simulink model "figure11_62"  (Simulink 7.1)
settings: Solver=ode3  StartTime=0.0  StopTime=20  MaxStep=0.001  MinStep=0.0000001  RelTol=1e-2  AbsTol=0.01
values from neighbouring files (symbols this model uses):
  dkd =     [fuzzpiddata.mat]
  dki =     [fuzzpiddata.mat]
  dkp =     [fuzzpiddata.mat]
settings Model: Creator=Administrator  LastModifiedBy=xierthy
settings DataIOCC: LimitDataPoints=off
settings OptimizationCC: InlineInvariantSignals=on
settings DebuggingCC: SaveWithParameterizedLinksMsg=none  SignalResolutionControl=TryResolveAllWithWarning  MultiTaskDSMMsg=warning  MultiTaskCondExecSysMsg=none  StrictBusMsg=None
settings RTWCC: IncludeERTFirstTime=on
settings GRTTargetCC: TargetFcnLib=ansi_tfl_tmw.mat

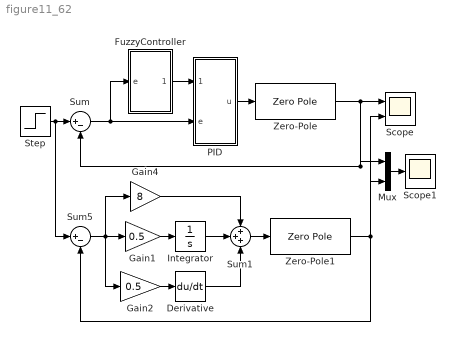
== system figure11_62 ==
  Derivative : Derivative
  FuzzyController : Subsystem
  Gain1 : Gain  Gain=0.5  ParameterDataType=sfix(16)  ParameterScaling=2^0  OutDataType=sfix(16)  OutScaling=2^0
  Gain2 : Gain  Gain=0.5  ParameterDataType=sfix(16)  ParameterScaling=2^0  OutDataType=sfix(16)  OutScaling=2^0
  Gain4 : Gain  Gain=8  ParameterDataType=sfix(16)  ParameterScaling=2^0  OutDataType=sfix(16)  OutScaling=2^0
  Integrator : Integrator
  Mux : Mux  Inputs=2
  PID : Subsystem
  Scope : Scope  NumInputPorts=2
      settings: TimeRange=20  YMin=1.00028~0.99525  YMax=1.00031~0.99555
  Scope1 : Scope
      settings: TimeRange=20  YMin=0.98  YMax=1.07  SaveName=ScopeData2
  Step : Step  Time=0  SampleTime=0
  Sum : Sum  Inputs=|+-  OutDataType=sfix(16)  OutScaling=2^0
  Sum1 : Sum  Inputs=+++  OutDataType=sfix(16)  OutScaling=2^0
  Sum5 : Sum  Inputs=|+-  OutDataType=sfix(16)  OutScaling=2^0
  Zero-Pole : ZeroPole  Zeros=[-0.5]  Poles=[-1 -1 -1]  Gain=[10]
  Zero-Pole1 : ZeroPole  Zeros=[-0.5]  Poles="[-1  -1 -1]"  Gain=[10]
  wires:
  Step/1 -> Sum/1, Sum5/1
  Sum/1 -> PID/2(e), FuzzyController/1(e)
  PID/1(u) -> Zero-Pole/1
  Zero-Pole/1 -> Scope/1, Sum/2, Mux/1
  FuzzyController/1(dPID) -> PID/1(dPID)
  Sum5/1 -> Gain1/1, Gain2/1, Gain4/1
  Gain2/1 -> Derivative/1
  Gain1/1 -> Integrator/1
  Integrator/1 -> Sum1/2
  Derivative/1 -> Sum1/3
  Zero-Pole1/1 -> Sum5/2, Scope/2, Mux/2
  Sum1/1 -> Zero-Pole1/1
  Gain4/1 -> Sum1/1
  Mux/1 -> Scope1/1

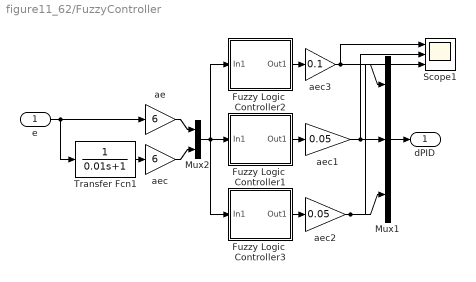
== system figure11_62/FuzzyController ==
  e : Inport  OutDataType=sfix(16)  OutScaling=2^0
  Fuzzy Logic  Controller1 : Subsystem  AncestorBlock="fuzblock/Fuzzy Logic  Controller"  mask(FIS){fis=dki}
      mask prompts: fis "FIS File or Structure:"
      mask help: FIS
      mask init:
      | fis = fuzblockmask(gcb,fis);
      mask Help: web(['file:///' docroot '/toolbox/fuzzy/fuzzylogiccontroller.html']);
      mask Display: plot(0, -0.3, 6, -0.3, 0, 1.2, 6, 1.2, [0 6], [0 0], [1 2 3],[0 1 0],[2 3 4],[0 1 0],[3 4 5],[0 1 0])
  Fuzzy Logic  Controller2 : Subsystem  AncestorBlock="fuzblock/Fuzzy Logic  Controller"  mask(FIS){fis=dkp}
      mask prompts: fis "FIS File or Structure:"
      mask help: FIS
      mask init:
      | fis = fuzblockmask(gcb,fis);
      mask Help: web(['file:///' docroot '/toolbox/fuzzy/fuzzylogiccontroller.html']);
      mask Display: plot(0, -0.3, 6, -0.3, 0, 1.2, 6, 1.2, [0 6], [0 0], [1 2 3],[0 1 0],[2 3 4],[0 1 0],[3 4 5],[0 1 0])
  Fuzzy Logic  Controller3 : Subsystem  AncestorBlock="fuzblock/Fuzzy Logic  Controller"  mask(FIS){fis=dkd}
      mask prompts: fis "FIS File or Structure:"
      mask help: FIS
      mask init:
      | fis = fuzblockmask(gcb,fis);
      mask Help: web(['file:///' docroot '/toolbox/fuzzy/fuzzylogiccontroller.html']);
      mask Display: plot(0, -0.3, 6, -0.3, 0, 1.2, 6, 1.2, [0 6], [0 0], [1 2 3],[0 1 0],[2 3 4],[0 1 0],[3 4 5],[0 1 0])
  Mux1 : Mux  Inputs=3
  Mux2 : Mux  Inputs=2
  Scope1 : Scope  NumInputPorts=3
      settings: TimeRange=10  YMin=-1~-0.5~-0.5  YMax=1~0.5~0.5
  Transfer Fcn1 : TransferFcn  Denominator=[0.01 1]
  ae : Gain  Gain=6  ParameterDataType=sfix(16)  ParameterScaling=2^0  OutDataType=sfix(16)  OutScaling=2^0
  aec : Gain  Gain=6  ParameterDataType=sfix(16)  ParameterScaling=2^0  OutDataType=sfix(16)  OutScaling=2^0
  aec1 : Gain  Gain=0.05  ParameterDataType=sfix(16)  ParameterScaling=2^0  OutDataType=sfix(16)  OutScaling=2^0
  aec2 : Gain  Gain=0.05  ParameterDataType=sfix(16)  ParameterScaling=2^0  OutDataType=sfix(16)  OutScaling=2^0
  aec3 : Gain  Gain=0.1  ParameterDataType=sfix(16)  ParameterScaling=2^0  OutDataType=sfix(16)  OutScaling=2^0
  dPID : Outport
  wires:
  Fuzzy Logic  Controller2/1(Out1) -> aec3/1
  Fuzzy Logic  Controller1/1(Out1) -> aec1/1
  Fuzzy Logic  Controller3/1(Out1) -> aec2/1
  e/1 -> ae/1, Transfer Fcn1/1
  Transfer Fcn1/1 -> aec/1
  ae/1 -> Mux2/1
  aec/1 -> Mux2/2
  Mux2/1 -> Fuzzy Logic  Controller1/1(In1), Fuzzy Logic  Controller3/1(In1), Fuzzy Logic  Controller2/1(In1)
  aec1/1 -> Mux1/2, Scope1/2
  aec2/1 -> Mux1/3, Scope1/3
  aec3/1 -> Mux1/1, Scope1/1
  Mux1/1 -> dPID/1

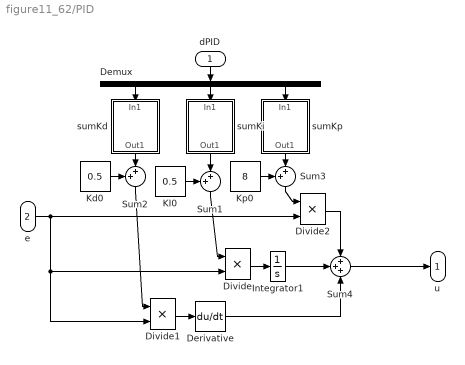
== system figure11_62/PID ==
  dPID : Inport  Orientation=down
  e : Inport  Port=2
  Demux : Demux  Orientation=down  Outputs=3
  Derivative : Derivative
  Divide : Product  Inputs=**  OutDataType=sfix(16)  OutScaling=2^-10
  Divide1 : Product  Inputs=**  OutDataType=sfix(16)  OutScaling=2^-10
  Divide2 : Product  Inputs=**  OutDataType=sfix(16)  OutScaling=2^-10
  Integrator1 : Integrator
  KI0 : Constant  Value=0.5  OutDataType=sfix(16)  OutScaling=2^0
  Kd0 : Constant  Value=0.5  OutDataType=sfix(16)  OutScaling=2^0
  Kp0 : Constant  Value=8  OutDataType=sfix(16)  OutScaling=2^0
  Sum1 : Sum  Orientation=down  Inputs=++|  OutDataType=sfix(16)  OutScaling=2^0
  Sum2 : Sum  Orientation=down  Inputs=++|  OutDataType=sfix(16)  OutScaling=2^0
  Sum3 : Sum  Orientation=down  Inputs=++|  OutDataType=sfix(16)  OutScaling=2^0
  Sum4 : Sum  Inputs=+++  OutDataType=sfix(16)  OutScaling=2^0
  sumKd : Subsystem  Orientation=down
  sumKi : Subsystem  Orientation=down
  sumKp : Subsystem  Orientation=down
  u : Outport  OutDataType=sfix(16)  OutScaling=2^0
  wires:
  Sum3/1 -> Divide2/1
  Sum2/1 -> Divide1/1
  Kp0/1 -> Sum3/1
  Kd0/1 -> Sum2/1
  KI0/1 -> Sum1/1
  Sum1/1 -> Divide/1
  e/1 -> Divide2/2, Divide/2, Divide1/2
  Divide2/1 -> Sum4/1
  Divide/1 -> Integrator1/1
  Divide1/1 -> Derivative/1
  Sum4/1 -> u/1
  dPID/1 -> Demux/1
  Demux/3 -> sumKp/1(In1)
  Demux/2 -> sumKi/1(In1)
  Demux/1 -> sumKd/1(In1)
  Integrator1/1 -> Sum4/2
  Derivative/1 -> Sum4/3
  sumKp/1(Out1) -> Sum3/2
  sumKi/1(Out1) -> Sum1/2
  sumKd/1(Out1) -> Sum2/2

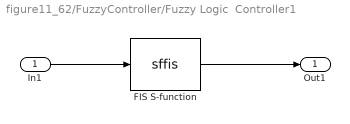
== system figure11_62/FuzzyController/Fuzzy Logic  Controller1 ==
  In1 : Inport  OutDataType=sfix(16)  OutScaling=2^0
  FIS S-function : S-Function  FunctionName=sffis  Parameters=fis  SFunctionModules=sfsup  EnableBusSupport=off
  Out1 : Outport  OutDataType=sfix(16)  OutScaling=2^0
  wires:
  FIS S-function/1 -> Out1/1
  In1/1 -> FIS S-function/1

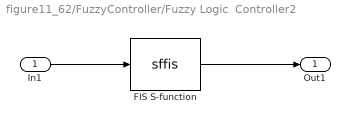
== system figure11_62/FuzzyController/Fuzzy Logic  Controller2 ==
  In1 : Inport  OutDataType=sfix(16)  OutScaling=2^0
  FIS S-function : S-Function  FunctionName=sffis  Parameters=fis  SFunctionModules=sfsup  EnableBusSupport=off
  Out1 : Outport  OutDataType=sfix(16)  OutScaling=2^0
  wires:
  In1/1 -> FIS S-function/1
  FIS S-function/1 -> Out1/1

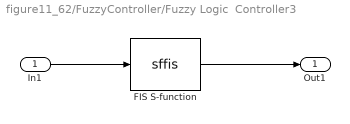
== system figure11_62/FuzzyController/Fuzzy Logic  Controller3 ==
  In1 : Inport  OutDataType=sfix(16)  OutScaling=2^0
  FIS S-function : S-Function  FunctionName=sffis  Parameters=fis  SFunctionModules=sfsup  EnableBusSupport=off
  Out1 : Outport  OutDataType=sfix(16)  OutScaling=2^0
  wires:
  In1/1 -> FIS S-function/1
  FIS S-function/1 -> Out1/1

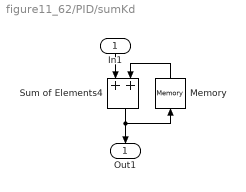
== system figure11_62/PID/sumKd ==
  In1 : Inport  Orientation=down
  Memory : Memory  Orientation=up  InheritSampleTime=on
  Sum of Elements4 : Sum  Orientation=down  OutDataType=sfix(16)  OutScaling=2^-10  SampleTime=0.001
  Out1 : Outport  Orientation=down
  wires:
  Sum of Elements4/1 -> Out1/1, Memory/1
  Memory/1 -> Sum of Elements4/2
  In1/1 -> Sum of Elements4/1

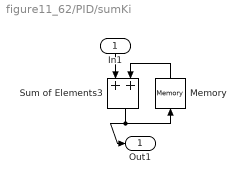
== system figure11_62/PID/sumKi ==
  In1 : Inport  Orientation=down
  Memory : Memory  Orientation=up  InheritSampleTime=on
  Sum of Elements3 : Sum  Orientation=down  OutDataType=sfix(16)  OutScaling=2^-10  SampleTime=0.001
  Out1 : Outport
  wires:
  Sum of Elements3/1 -> Out1/1, Memory/1
  Memory/1 -> Sum of Elements3/2
  In1/1 -> Sum of Elements3/1

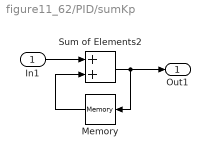
== system figure11_62/PID/sumKp ==
  In1 : Inport
  Memory : Memory  Orientation=left  InheritSampleTime=on
  Sum of Elements2 : Sum  OutDataType=sfix(16)  OutScaling=2^-10  SampleTime=0.001
  Out1 : Outport
  wires:
  In1/1 -> Sum of Elements2/1
  Memory/1 -> Sum of Elements2/2
  Sum of Elements2/1 -> Out1/1, Memory/1
